simulink model "Conventional_MPC_10khz_DEMO1"  (R2022b)
settings: Solver=VariableStepAuto  StartTime=0.0  StopTime=0.04  FixedStep=1e-07  MaxStep=1e-4  RelTol=1e-3
libraries: spsIGBTDiodeLib x12, spsSeriesRLCBranchLib x7, spsVoltageMeasurementLib x4, spsCurrentMeasurementLib x3, spsDCVoltageSourceLib x2, spsTHDLib x2, spsSawtoothGeneratorLib x1, spsabctoAlphaBetaZeroLib x1, spspowerguiLib x1
settings Model: Creator=khoap  LastModifiedBy=DELL
settings SolverCC: AlgebraicLoopSolver=TrustRegion
settings DataIOCC: ReturnWorkspaceOutputs=off
settings DebuggingCC: UnconnectedInputMsg=warning  UnconnectedOutputMsg=warning  UnconnectedLineMsg=warning  SFMachineParentedDataDiag=warning  ArithmeticOperatorsInVariantConditions=warning
settings ModelReferenceCC: EnableRefExpFcnMdlSchedulingChecks=on
settings SFSimCC: SimUseLocalCustomCode=off  CustomCodeUndefinedFunction=UseInterfaceOnly
settings RTWCC: RTWUseLocalCustomCode=off
settings CodeAppCC: StateflowObjectComments=on

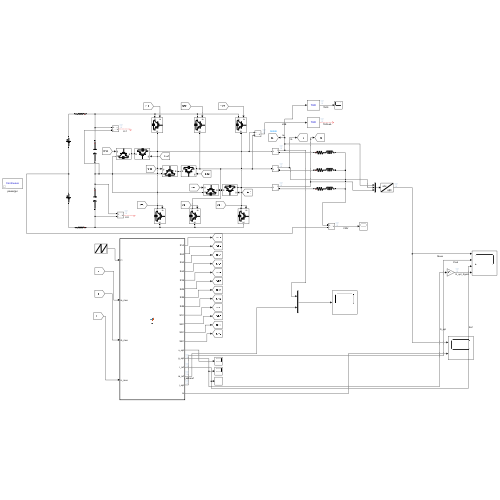
[thumbnail: Simulink's stored preview of the top-level diagram]
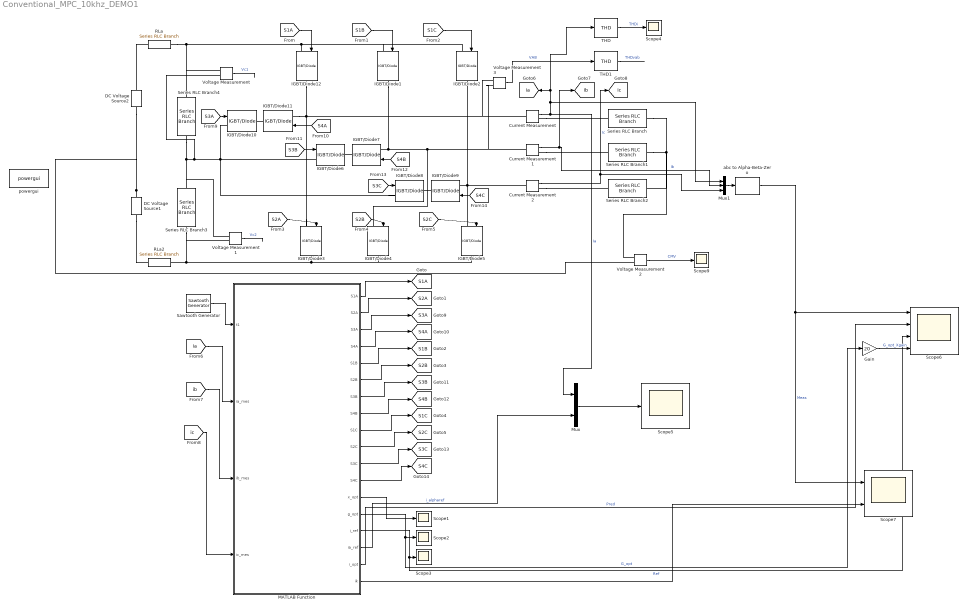
== system Conventional_MPC_10khz_DEMO1 ==
  Current Measurement : spsCurrentMeasurementLib/Current Measurement  PhasorSimulation=off  OutputType=Complex  PSBequivalent=0
  Current Measurement1 : spsCurrentMeasurementLib/Current Measurement  PhasorSimulation=off  OutputType=Complex  PSBequivalent=0
  Current Measurement2 : spsCurrentMeasurementLib/Current Measurement  PhasorSimulation=off  OutputType=Complex  PSBequivalent=0
  DC Voltage Source1 : spsDCVoltageSourceLib/DC Voltage Source  Amplitude=100  Measurements=None
  DC Voltage Source2 : spsDCVoltageSourceLib/DC Voltage Source  Amplitude=100  Measurements=None
  Gain : Gain  Gain=20
  IGBT/Diode{1..12} (12 alike) : spsIGBTDiodeLib/IGBT//Diode  Ron=1e-3  Rs=1e5  Cs=inf  Measurements=off
  MATLAB Function : MATLAB Function  TreatAsAtomicUnit=on
  Mux : Mux  Inputs=2
  Mux1 : Mux  Inputs=3
  RLa : spsSeriesRLCBranchLib/Series RLC Branch  LConnTagsString=__new0  RConnTagsString=__new0  BranchType=R  Resistance=0.001  Inductance=0.05  SetiL0=off  InitialCurrent=0  Capacitance=1.0  Setx0=off  InitialVoltage=0  Measurements=None
  RLa2 : spsSeriesRLCBranchLib/Series RLC Branch  LConnTagsString=__new0  RConnTagsString=__new0  BranchType=R  Resistance=0.001  Inductance=0.05  SetiL0=off  InitialCurrent=0  Capacitance=1.0  Setx0=off  InitialVoltage=0  Measurements=None
  Sawtooth Generator : spsSawtoothGeneratorLib/Sawtooth Generator  Freq=50  Phase=0  Ts=1/10000
  Scope{1..5,9} (6 alike) : Scope
  Scope6 : Scope  NumInputPorts=4
  Scope7 : Scope  NumInputPorts=2
  Series RLC Branch : spsSeriesRLCBranchLib/Series RLC Branch  LConnTagsString=__new0  RConnTagsString=__new0  BranchType=RL  Resistance=25  Inductance=50e-03  SetiL0=off  InitialCurrent=0  Capacitance=1e-6  Setx0=off  InitialVoltage=0  Measurements=None
  Series RLC Branch1 : spsSeriesRLCBranchLib/Series RLC Branch  LConnTagsString=__new0  RConnTagsString=__new0  BranchType=RL  Resistance=25  Inductance=50e-03  SetiL0=off  InitialCurrent=0  Capacitance=1e-6  Setx0=off  InitialVoltage=0  Measurements=None
  Series RLC Branch2 : spsSeriesRLCBranchLib/Series RLC Branch  LConnTagsString=__new0  RConnTagsString=__new0  BranchType=RL  Resistance=25  Inductance=50e-03  SetiL0=off  InitialCurrent=0  Capacitance=1e-6  Setx0=off  InitialVoltage=0  Measurements=None
  Series RLC Branch3 : spsSeriesRLCBranchLib/Series RLC Branch  LConnTagsString=__new0  RConnTagsString=__new0  BranchType=C  Resistance=1  Inductance=1e-3  SetiL0=off  InitialCurrent=0  Capacitance=3300e-6  Setx0=on  InitialVoltage=100  Measurements=None
  Series RLC Branch4 : spsSeriesRLCBranchLib/Series RLC Branch  LConnTagsString=__new0  RConnTagsString=__new0  BranchType=C  Resistance=1  Inductance=1e-3  SetiL0=off  InitialCurrent=0  Capacitance=3300e-6  Setx0=on  InitialVoltage=100  Measurements=None
  THD : spsTHDLib/THD  Freq=50  Ts=10e-8
  THD1 : spsTHDLib/THD  Freq=50  Ts=10e-8
  Voltage Measurement{,1..3} (4 alike) : spsVoltageMeasurementLib/Voltage Measurement  PhasorSimulation=off  OutputType=Complex  PSBequivalent=0
  abc to Alpha-Beta-Zero : spsabctoAlphaBetaZeroLib/abc to Alpha-Beta-Zero
  powergui : spspowerguiLib/powergui  Priority=1  SimulationMode=Continuous  SampleTime=1e-07  frequency=60  Iterations=50  frequencyindice=0  Pbase=100e6  ErrMax=1e-4  UnitsV=kV  UnitsW=MW  buscounter=0  FunctionMessages=off  echomessages=off  EnableUseOfTLC=off  CurrentSourceSwitches=off  DisableSnubberDevices=off  DisableRonSwitches=off  DisableVfSwitches=off  DisplayEquations=off  AutomaticDiscreteSolvers=off  SolverType=Tustin/Backward Euler (TBE)  Interpol=off  ExternalGateDelay=off  methode=off  Ts=100  x0status=blocks  SPID=on  SwTol=0  HookPort=off  NonlinearTolerance=1e-4  nMaxIteration=100  ContinueOnMaxIteration=off  RestoreLinks=warning  ResistiveCurrentMeasurement=off  Frange=[0:2:500]  Ylog=off  Xlog=on  ShowGrid=off  save=off  variable=ZData  structure=0  ZoomFFT=off  StartTime=0.0  cycles=1  DisplayStyle=1  fundamental=60  FreqAxis=off  MaxFrequency=1000  frequencyindicesteady=1  RmsSteady=1  display=off
  tag scope: S1A=global, S1B=global, S1C=global, S2A=global, S2B=global, S2C=global, S3A=global, S3B=global, S3C=global, S4A=global, S4B=global, S4C=global, ia=global, ib=global, ic=global
  wires:
  [S1A] -> IGBT/Diode12/1
  [S1B] -> IGBT/Diode1/1
  [S1C] -> IGBT/Diode2/1
  [S2A] -> IGBT/Diode3/1
  [S2B] -> IGBT/Diode4/1
  [S2C] -> IGBT/Diode5/1
  Sawtooth Generator/1 -> MATLAB Function/1(t1)
  MATLAB Function/2(S2A) -> [S2A]
  MATLAB Function/5(S1B) -> [S1B]
  MATLAB Function/6(S2B) -> [S2B]
  MATLAB Function/9(S1C) -> [S1C]
  MATLAB Function/10(S2C) -> [S2C]
  Current Measurement1/1 -> Mux1/2, [ib]  "Ib"
  Current Measurement2/1 -> Mux1/3, [ic]  "Ic"
  [ia] -> MATLAB Function/2(ia_mes)
  [ib] -> MATLAB Function/3(ib_mes)
  [ic] -> MATLAB Function/4(ic_mes)
  MATLAB Function/1(S1A) -> [S1A]
  Current Measurement/1 -> Mux1/1, THD/1, [ia], Mux/1  "Ia"
  Mux/1 -> Scope5/1
  MATLAB Function/16(ia_ref) -> Mux/2  "i_alpharef"
  MATLAB Function/7(S3B) -> [S3B]
  MATLAB Function/8(S4B) -> [S4B]
  MATLAB Function/3(S3A) -> [S3A]
  MATLAB Function/4(S4A) -> [S4A]
  MATLAB Function/11(S3C) -> [S3C]
  MATLAB Function/12(S4C) -> [S4C]
  [S3A] -> IGBT/Diode10/1
  [S4A] -> IGBT/Diode11/1
  [S3B] -> IGBT/Diode6/1
  [S4B] -> IGBT/Diode7/1
  [S3C] -> IGBT/Diode8/1
  [S4C] -> IGBT/Diode9/1
  MATLAB Function/15(i_ref) -> Scope3/1, Scope6/3  "Ref"
  THD/1 -> Scope4/1  "THDi"
  Mux1/1 -> abc to Alpha-Beta-Zero/1
  abc to Alpha-Beta-Zero/1 -> Scope7/1, Scope6/1  "Meas"
  MATLAB Function/17(i_opt) -> Scope6/2  "Pred"
  MATLAB Function/18(ik) -> Scope7/2
  MATLAB Function/14(g_opt) -> Gain/1, Scope2/1  "G_opt"
  Gain/1 -> Scope6/4  "G_opt_Xgain"
  MATLAB Function/13(x_opt) -> Scope1/1
  Voltage Measurement2/1 -> Scope9/1  "CMV"
  THD1/1 -> ?  "THDvab"
  Voltage Measurement3/1 -> THD1/1  "VAB"
  Voltage Measurement/1 -> ?  "Vc1"
  Voltage Measurement1/1 -> ?  "Vc2"
  connections:
  IGBT/Diode2/LConn1 -- IGBT/Diode1/LConn1 -- Voltage Measurement/LConn1 -- Series RLC Branch4/LConn1 -- RLa/LConn1 -- IGBT/Diode12/LConn1
  IGBT/Diode5/LConn1 -- Current Measurement2/LConn1 -- IGBT/Diode2/RConn1 -- IGBT/Diode9/LConn1
  IGBT/Diode4/LConn1 -- IGBT/Diode1/RConn1 -- IGBT/Diode7/LConn1 -- Voltage Measurement3/LConn2 -- Current Measurement1/LConn1
  IGBT/Diode3/LConn1 -- Voltage Measurement3/LConn1 -- Current Measurement/LConn1 -- IGBT/Diode12/RConn1 -- IGBT/Diode11/LConn1
  IGBT/Diode3/RConn1 -- IGBT/Diode5/RConn1 -- IGBT/Diode4/RConn1 -- Series RLC Branch3/RConn1 -- Voltage Measurement1/LConn2 -- RLa2/LConn1
  Series RLC Branch/RConn1 -- Voltage Measurement2/LConn1 -- Series RLC Branch2/RConn1 -- Series RLC Branch1/RConn1
  Current Measurement/RConn1 -- Series RLC Branch/LConn1
  Current Measurement1/RConn1 -- Series RLC Branch1/LConn1
  Current Measurement2/RConn1 -- Series RLC Branch2/LConn1
  IGBT/Diode7/RConn1 -- IGBT/Diode6/RConn1
  IGBT/Diode9/RConn1 -- IGBT/Diode8/RConn1
  IGBT/Diode10/RConn1 -- IGBT/Diode11/RConn1
  DC Voltage Source1/LConn1 -- RLa2/RConn1
  DC Voltage Source2/RConn1 -- RLa/RConn1
  DC Voltage Source1/RConn1 -- Voltage Measurement2/LConn2 -- DC Voltage Source2/LConn1
  IGBT/Diode8/LConn1 -- IGBT/Diode6/LConn1 -- IGBT/Diode10/LConn1 -- Voltage Measurement/LConn2 -- Voltage Measurement1/LConn1 -- Series RLC Branch3/LConn1 -- Series RLC Branch4/RConn1

== matlab function Conventional_MPC_10khz_DEMO1/MATLAB Function ==
  settings: updateMethod=DISCRETE
  data: t1 input; S1A output; S2A output; S3A output; S4A output; S1B output; S2B output; S3B output; S4B output; S1C output; S2C output; S3C output; S4C output; ia_mes input; ib_mes input; ic_mes input; x_opt output size=1; g_opt output size=1; i_ref output; ia_ref output; i_opt output; ik output
function [S1A,S2A,S3A, S4A, S1B,S2B, S3B, S4B, S1C,S2C, S3C, S4C, x_opt,g_opt,i_ref,ia_ref, i_opt,ik]  = fcn(t1,ia_mes,ib_mes,ic_mes)
t = (t1+1)/100;
Ts = 1/10000;
R = 25;
L = 50e-03;
w = 2*pi*50;
Vdc = 200;
C = 3300e-6;
I_ref_peak = 2;
ia_ref = I_ref_peak*cos(w*t);
ib_ref = I_ref_peak*cos(w*t - 2*pi/3);
ic_ref = I_ref_peak*cos(w*t - 4*pi/3);
a = cos(2*pi/3)+1i*sin(2*pi/3);
aa = cos(4*pi/3)+1i*sin(4*pi/3);
i_ref = (2/3)*(ia_ref + ib_ref*a + ic_ref*aa);
ik = (2/3)*(ia_mes + ib_mes*a + ic_mes*aa);

v0 = 0;
v1 = (2/3)*(1/2)*Vdc;
v2 = (2/3)*(1)*Vdc;
v3 = (2/3)*(a/2)*Vdc;
v4 = (2/3)*(1/2 + a/2)*Vdc;
v5 = (2/3)*(1 + a/2)*Vdc;
v6 = (2/3)*(a)*Vdc;
v7 = (2/3)*(1/2 + a)*Vdc;
v8 = (2/3)*(1 + a)*Vdc;
v9 = (2/3)*(aa/2)*Vdc;
v10 = (2/3)*(aa/2 + 1/2)*Vdc;
v11 = (2/3)*(aa/2 + 1)*Vdc;
v12 = (2/3)*(aa/2 + a/2)*Vdc;
v13 = (2/3)*(aa/2 + 1/2 + a/2)*Vdc;
v14 = (2/3)*(aa/2 + 1 + a/2)*Vdc;
v15 = (2/3)*(aa/2 + a)*Vdc;
v16 = (2/3)*(aa/2 + 1/2 + a)*Vdc;
v17 = (2/3)*(aa/2 + 1 + a)*Vdc;
v18 = (2/3)*(aa)*Vdc;
v19 = (2/3)*(aa + 1/2)*Vdc;
v20 = (2/3)*(aa + 1)*Vdc;
v21 = (2/3)*(aa + a/2)*Vdc;
v22 = (2/3)*(aa + 1/2 + a/2)*Vdc;
v23 = (2/3)*(aa + 1 + a/2)*Vdc;
v24 = (2/3)*(aa + a)*Vdc;
v25 = (2/3)*(aa + 1/2 + a)*Vdc;
v26 = 0;

v = [v0 v1 v2 v3 v4 v5 v6 v7 v8 v9 v10 v11 v12 v13 v14 v15 v16 v17 v18 v19 v20 v21 v22 v23 v24 v25 v26];
states = [0 0 0 0 0 0; 0 0 0 0 0 1; 0 0 0 0 1 1; 0 0 0 1 0 0; 0 0 0 1 0 1; 0 0 0 1 1 1; 0 0 1 1 0 0; 0 0 1 1 0 1; 0 0 1 1 1 1;
          0 1 0 0 0 0; 0 1 0 0 0 1; 0 1 0 0 1 1; 0 1 0 1 0 0; 0 1 0 1 0 1; 0 1 0 1 1 1; 0 1 1 1 0 0; 0 1 1 1 0 1; 0 1 1 1 1 1;
          1 1 0 0 0 0; 1 1 0 0 0 1; 1 1 0 0 1 1; 1 1 0 1 0 0; 1 1 0 1 0 1; 1 1 0 1 1 1; 1 1 1 1 0 0; 1 1 1 1 0 1; 1 1 1 1 1 1;];
g_opt = 10e09;
g_opt1 = 0;
x_opt1 = 0;
i_opt = 0 + 1i*0;

% vc1_k1 = Vc1 + i/2/C*Ts; 
% vc2_k1 = Vc2 + ic2/2/C*Ts; 
for i = 1:27
    ip_k1 = (1 - R*Ts/L)*ik + (Ts/L)*v(i); 
    g = abs(real(i_ref - ip_k1)) + abs(imag(i_ref - ip_k1));
    if(g <= g_opt)
        g_opt = g;
        x_opt = i;
        g_opt1 = g_opt;
        x_opt1 = x_opt;
        i_opt = ip_k1;
    else
        g_opt = g_opt1;
        x_opt = x_opt1;
    end
end
S1A = states(x_opt,5);
S1B = states(x_opt,3);
S1C = states(x_opt,1);
S4A = not(S1A);
S4B = not(S1B);
S4C = not(S1C);
S3A = states(x_opt,6);
S3B = states(x_opt,4);
S3C = states(x_opt,2);
S2A = not(S3A);
S2B = not(S3B);
S2C = not(S3C);
end
